simulink model "J545"  (R2015b)
settings: Solver=VariableStepAuto  StartTime=-10  StopTime=10.0  RelTol=1e-3
libraries: simulink x1
settings Model: Creator=Pouya  LastModifiedBy=Pouya

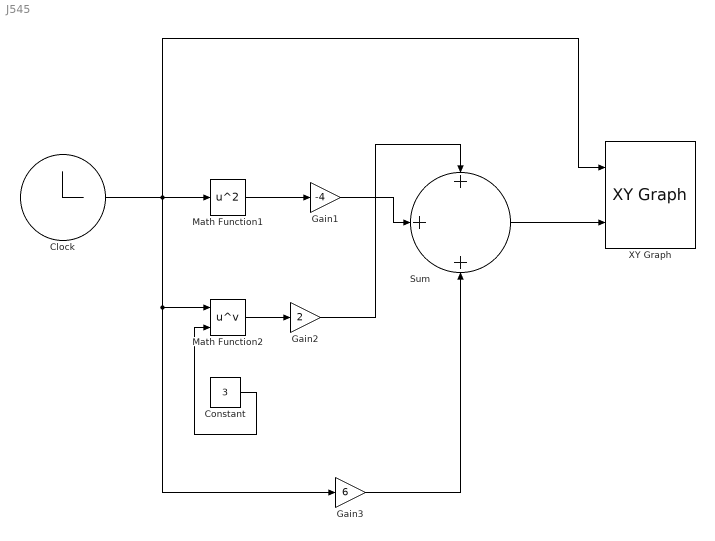
== system J545 ==
  Clock : Clock
  Constant : Constant  Value=3
  Gain1 : Gain  Gain=-4
  Gain2 : Gain  Gain=2
  Gain3 : Gain  Gain=6
  Math Function1 : Math  Operator=square  SaturateOnIntegerOverflow=on
  Math Function2 : Math  Operator=pow  SaturateOnIntegerOverflow=on
  Sum : Sum  Inputs=+++
  XY Graph : simulink/Sinks/XY Graph  xmin=-10  xmax=10  ymin=-100  ymax=100  st=-1
  wires:
  Clock/1 -> Math Function1/1, Gain3/1, Math Function2/1, XY Graph/1
  Constant/1 -> Math Function2/2
  Math Function2/1 -> Gain2/1
  Math Function1/1 -> Gain1/1
  Sum/1 -> XY Graph/2
  Gain2/1 -> Sum/1
  Gain1/1 -> Sum/2
  Gain3/1 -> Sum/3
